simulink library "INT_EngPrt_OvrSpd"  (R2016b)
settings: Solver=VariableStepAuto  StartTime=0.0  StopTime=10.0  RelTol=1e-3
settings Model: Creator=Administrator  LastModifiedBy=Administrator

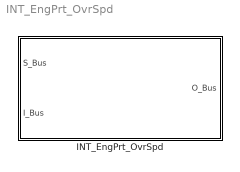
== system INT_EngPrt_OvrSpd ==
  INT_EngPrt_OvrSpd : Subsystem

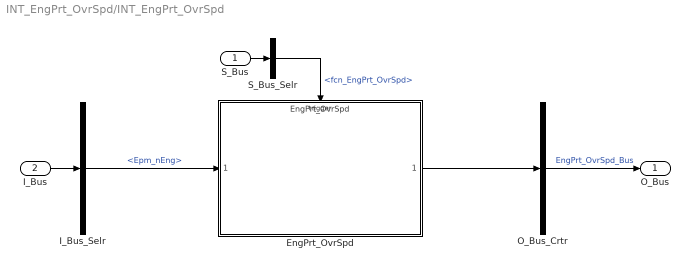
== system INT_EngPrt_OvrSpd/INT_EngPrt_OvrSpd ==
  S_Bus : Inport
  I_Bus : Inport  Port=2
  EngPrt_OvrSpd : ModelReference  ModelNameDialog=EngPrt_OvrSpd  SimulationMode=Normal  ModelReferenceVersion=1.7  TriggerPortName=function  TriggerPortTriggerType=function-call  TriggerPortStatesWhenEnabling=held
  I_Bus_Selr : BusSelector  OutputSignals=Epm_nEng
  O_Bus_Crtr : BusCreator  Inputs=1
  S_Bus_Selr : BusSelector  OutputSignals=fcn_EngPrt_OvrSpd
  O_Bus : Outport
  wires:
  S_Bus_Selr/1 -> EngPrt_OvrSpd/Trigger  "<fcn_EngPrt_OvrSpd>"
  S_Bus/1 -> S_Bus_Selr/1
  I_Bus/1 -> I_Bus_Selr/1
  I_Bus_Selr/1 -> EngPrt_OvrSpd/1  "<Epm_nEng>"
  O_Bus_Crtr/1 -> O_Bus/1  "EngPrt_OvrSpd_Bus"
  EngPrt_OvrSpd/1 -> O_Bus_Crtr/1
